simulink model "Laboratory_3_Deboucing"  (R2023b)
settings: Solver=FixedStepDiscrete  StartTime=0.0  StopTime=10  FixedStep=0.01  RelTol=1e-3
libraries: SignalEditorBlockLib x1
settings Model: Creator=cosmi  LastModifiedBy=cosmi

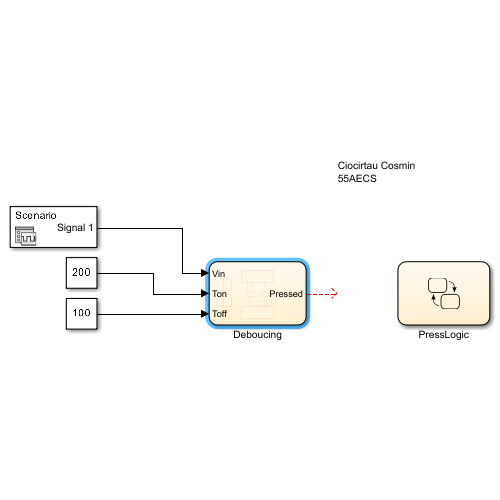
[thumbnail: Simulink's stored preview of the top-level diagram]
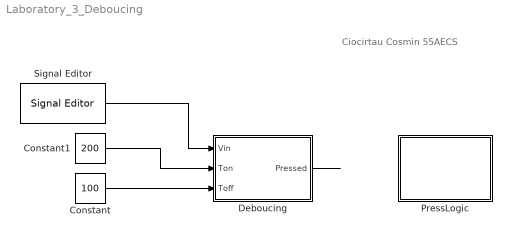
== system Laboratory_3_Deboucing ==
  note: Ciocirtau Cosmin
      | 55AECS
  Constant : Constant  Value=100
  Constant1 : Constant  Value=200
  Deboucing : Stateflow chart  TreatAsAtomicUnit=on
  PressLogic : Stateflow chart  TreatAsAtomicUnit=on
  Signal Editor : SignalEditorBlockLib/Signal Editor  FileName=E:\Matlab & Simulink\ESDM\signal_lab3.mat  ActiveScenario=Scenario  ActiveSignal=Signal 1  IsBus=off  OutputBusObjectStr=Bus: BusObject  SampleTime=0  Interpolate=off  ZeroCross=off  OutputAfterFinalValue=Setting to zero  Unit=inherit  PreserveSignalName=on  ApplySigPropsToAllScenarios=on  ApplySigPropsToAllSignals=off
  wires:
  Constant/1 -> Deboucing/3(Toff)
  Constant1/1 -> Deboucing/2(Ton)
  Signal Editor/1 -> Deboucing/1(Vin)
  Deboucing/1(Pressed) -> ?

== stateflow chart Laboratory_3_Deboucing/PressLogic ==

== stateflow chart Laboratory_3_Deboucing/Deboucing ==
  state NOT_PRESSED
    en:
    Output = false;
  note: Inputs:
      | -Vin
      |
      | Outputs:
      | -Pressed
  state Just to make things [group]
    look nice. :D
  state WAIT1
  state WAIT2
  state Ciocirtau Cosmin [group]
    55AECS
  state PRESSED
    en:
    Output = true;
  (default) -> NOT_PRESSED
  NOT_PRESSED -> WAIT1 : [Input == true]
  WAIT1 -> NOT_PRESSED [order 2] : [Input == false]
  WAIT2 -> NOT_PRESSED [order 2] : [after(T_off, sec)]
  WAIT1 -> PRESSED [order 1] : [after(T_on, sec)]
  PRESSED -> WAIT2 : [Input == false]
  WAIT2 -> PRESSED [order 1] : [Input == true]
  data: Vin input; Ton input; Toff input; Pressed output
